simulink model "Question4_Model"  (R2019b)
settings: Solver=VariableStepAuto  StartTime=0.0  StopTime=10.0  RelTol=1e-3
settings Model: Creator=EASY LIFE  LastModifiedBy=EASY LIFE

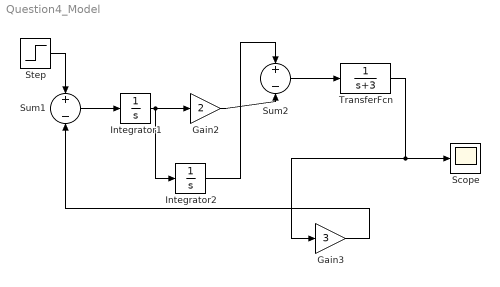
== system Question4_Model ==
  Gain2 : Gain  Gain=2
  Gain3 : Gain  Gain=3
  Integrator1 : Integrator
  Integrator2 : Integrator
  Scope : Scope
  Step : Step  SampleTime=0
  Sum1 : Sum  Inputs=+-
  Sum2 : Sum  Inputs=+-
  TransferFcn : TransferFcn  Numerator=1  Denominator=[1 3]
  wires:
  Step/1 -> Sum1/1
  Sum1/1 -> Integrator1/1
  Integrator1/1 -> Gain2/1, Integrator2/1
  Gain2/1 -> Sum2/2
  Integrator2/1 -> Sum2/1
  Sum2/1 -> TransferFcn/1
  TransferFcn/1 -> Scope/1, Gain3/1
  Gain3/1 -> Sum1/2
